simulink model "Sim_Multi"  (R2023a)
settings: Solver=FixedStepAuto  StartTime=0.0  StopTime=20  FixedStep=t_sim  MaxStep=t_control  RelTol=1e-5  EnableMultiTasking=on
InitFcn:
  | %--------------------------------------------------------------------------
  | %% Multirotor Dynamic Simulation Environment for the Testing of GNC Algorithms
  | % This simulation is part of the Master's thesis titled
  | % "A Modular Simulation Environment for the Improved Dynamic Simulation of
  | % Multirotor Unmanned Aerial Vehicles",
  | % submitted to the University of Illinois at Urbana-Champaign in May 2016.
  | % The thesis itself can be found here: http://hdl.handle.net/2142/90660
  | % Jan Vervoorst, vervoors@illinois.edu
  | % University of Illinois 2015/16
  | %--------------------------------------------------------------------------
  | %% Initialization routine for the Simulink simulation file Sim_Multi.slx
  | %--------------------------------------------------------------------------
  | clear all;close all;clc
  | %--------------------------------------------------------------------------
  | t_control = 1/500;          % Controller/state estimation frequency 500Hz [s]
  | t_sim = t_control/2;        % Simulation frequency 1000Hz [s]
  | sim_time = 10.0;            % Duration of simulation [sec]
  | r2d = 180/pi;               % Conversion factor radians to degrees [deg/rad]
  | d2r = pi/180;               % Conversion factor degrees to radians [rad/deg]
  | g = 9.80665;                % Acceleration of gravity [m/s^2]
  | rpm2radpersec = 2*pi/60;    % Conversion factor RPM to rad/sec [rad/(s*rpm)]
  | rho = 1.225;                % Density of air [kg/m^3]
  | %--------------------------------------------------------------------------
  | %%%%%%%%%%%%%%%%%%%%%%%%%%%%%%%%%%%%%%%%%%%%%%%%%%%%%%%%%%%%%%%%%%%%%%%%%%%
  | %               Quad specific configuration parameters                    %
  | %%%%%%%%%%%%%%%%%%%%%%%%%%%%%%%%%%%%%%%%%%%%%%%%%%%%%%%%%%%%%%%%%%%%%%%%%%%
  | % The coordinate system used in this model is defined as follows:
  | % X: pointing forward, Roll axis
  | % Y: pointing to the right, Pitch axis
  | % Z: pointing down, Yaw axis
  | % To define the geometry of the airframe, the following convention is used:
  | % - the base airframe is assumed to be somewhat symmetric
  | % - the CoG for the base airframe coincides with the geometric center in X/Y plane (but is shifted along Z axis)
  | % - the motor arm length in X/Y plane is defined as the distance to the geometric center of the base airframe
  | % - motor thrust is generated at the prop, which is offset a distance (along Z) from the geometric center
  | % - motor thrust vector may be misaligned from purely Z direction, so a set of rotation angles is given for each motor
  | % - real position of CoG is given as a position vector from geometric center
  | % - everything is expressed in body coordinate system described above
  | %%%%%%%%%%%%%%%%%%%%%%%%%%%%%%%%%%%%%%%%%%%%%%%%%%%%%%%%%%%%%%%%%%%%%%%%%%%
  | Noise_flag = 0;                 % Set to 1 for sensor/estimation noise, to 0 for no noise
  | Coriolis_correction = 1;        % Set to 1 to cancel omega x (J*omega) term in control law, 0 if not
  | Dyn_thrust = 1;                 % Set to 1 to engage dynamic thrust effects, to 0 to disengage
  | Blade_flapping = 1;             % Set to 1 to engage blade flapping effects, to 0 to disengage
  | %%%%%%%%%%%%%%%%%%%%%%%%%%%%%%%%
  | % Initial conditions
  | Att_init = [0;0;0] * d2r;       % Initial airframe attitude in Euler angles Roll/Pitch/Yaw for 6DOF block [deg]
  | omega_init = [0;0;0];           % Initial angular rates in Body frame for 6DOF block [rad/s]
  | Vb_init = [0;0;0];              % Initial velocity in Body frame for 6DOF block [m/s]
  | Xi_init = [0;0;0];              % Initial position in Inertial frame for 6DOF block [m]
  | rpm_init = 3104.5025852;        % Initial motor speed [rpm]
  | q_init = rpy2quat(Att_init);    % Compute the initial attitude quaternion
  | R_IB_init = rpy2rot(Att_init);  % Compute the initial rotation matrix R_IB
  | Vi_init = R_IB_init' * Vb_init; % Compute the initial velocity in Inertial axes
  | %%%%%%%%%%%%%%%%%%%%%%%%%%%%%%%%
  | % Parameters for aerodynamic drag computation
  | a = 0.060;                      % Surface area of airframe visible along the Body x axis [m^2]
  | b = 0.060;                      % Surface area of airframe visible along the Body y axis [m^2]
  | c = 0.060;                      % Surface area of airframe visible along the Body z axis [m^2]
  | C_D = 0.40;                     % Drag coefficient [dimensionless]
  | Surface_params = [a;b;c];       % Combine the surface area parameters
  | ... (+145 lines)
undefined symbols (not defined in the file or in its folder): DiscIntNeverNeededParam, rpy2quat, thrust2rpm
libraries: simulink x20
(part 3 of 4)

== system Sim_Multi/multirotor/Force//Moment computation/Forces and moments generated by spinning propellers/For Each Subsystem/Leverarm vector from real CoG to each propeller (Body axes) ==
  note: This subsystem computes the leverarm vector from the real center of gravity
      | of the airframe to each propeller.
      | This vector is necessary to compute the moment contributions of each propeller.
  MotorMatrix_real : Inport
  CoG_real : Inport  Port=2
  Abs : Abs  SaturateOnIntegerOverflow=off
  Conversion deg to rad : Gain  Gain=d2r
  Mux : Mux  Inputs=2
  Mux2 : Mux  Inputs=2
  Product4 : Product
  Reshape : Reshape  OutputDimensionality=Column vector (2-D)
  Reshape1 : Reshape  OutputDimensionality=Column vector (2-D)
  Selector3 : Selector  InputPortWidth=17  IndexOptions=Index vector (dialog)  Indices=[1]  OutputSizes=1
  Selector4 : Selector  InputPortWidth=17  IndexOptions=Index vector (dialog)  Indices=[2]  OutputSizes=1
  Selector5 : Selector  InputPortWidth=17  IndexOptions=Index vector (dialog)  Indices=[3]  OutputSizes=1
  Subtract : Sum  Inputs=+-
  Trigonometric Function : Trigonometry
  Trigonometric Function1 : Trigonometry  Operator=cos
  Prop_vector : Outport
  wires:
  Selector3/1 -> Conversion deg to rad/1  "Motor arm angle"
  Selector4/1 -> Abs/1  "Motor arm length"
  Selector5/1 -> Mux2/2  "Propeller Z offset"
  Conversion deg to rad/1 -> Trigonometric Function/1, Trigonometric Function1/1
  Trigonometric Function1/1 -> Mux/1  "Motor arm x component"
  Trigonometric Function/1 -> Mux/2  "Motor arm y component"
  Mux/1 -> Product4/1
  Abs/1 -> Product4/2
  Product4/1 -> Mux2/1  "Motor location x/y vector"
  Mux2/1 -> Reshape/1
  CoG_real/1 -> Reshape1/1  "Location of real CoG w.r.t. geometric center (Body axes)"
  Reshape/1 -> Subtract/1  "Vector from geometric center to propeller (Body axes)"
  Reshape1/1 -> Subtract/2
  Subtract/1 -> Prop_vector/1  "Vector from real CoG to propeller (Body axes)"
  MotorMatrix_real/1 -> Selector5/1, Selector4/1, Selector3/1

== system Sim_Multi/multirotor/Force//Moment computation/Forces and moments generated by spinning propellers/For Each Subsystem/Thrust//moment vector for each propeller (Body axes) ==
  Prop_vector : Inport
  True airspeed : Inport  Port=2
  Body_rates : Inport  Port=3
  MotorMatrix_real : Inport  Port=4
  RPM_motor : Inport  Port=5
  Add : Sum  Inputs=++++
  Compute dynamic motor thrust and moments : Subsystem
  Coordinate transformation Body to Motor axes : Subsystem
  Cross Product : Subsystem
  Reshape : Reshape  OutputDimensionality=Column vector (2-D)
  Thrust_vector (Body axes) : Outport
  Motor_moments (Body axes) : Outport  Port=2
  wires:
  MotorMatrix_real/1 -> Coordinate transformation Body to Motor axes/1(MotorMatrix_real), Compute dynamic motor thrust and moments/2(MotorMatrix_real)
  True airspeed/1 -> Coordinate transformation Body to Motor axes/2(Airspeed (Body axes))
  Coordinate transformation Body to Motor axes/2(Airspeed (Motor axes)) -> Compute dynamic motor thrust and moments/4(Airspeed (Motor axes))
  RPM_motor/1 -> Compute dynamic motor thrust and moments/1(RPM_motor)
  Body_rates/1 -> Compute dynamic motor thrust and moments/5(Body_rates)
  Compute dynamic motor thrust and moments/3(Gyro moment (Body axes)) -> Add/3  "Gyroscopic moments per motor (Body axes)"
  Compute dynamic motor thrust and moments/1(Induced motor moment (Body axes)) -> Add/1  "Induced motor moment at dynamic conditions (Body axes)"
  Add/1 -> Motor_moments (Body axes)/1
  Coordinate transformation Body to Motor axes/1(R_mb) -> Compute dynamic motor thrust and moments/3(R_mb)
  Compute dynamic motor thrust and moments/4(Thrust_vector (Body axes)) -> Thrust_vector (Body axes)/1, Cross Product/2(v)
  Compute dynamic motor thrust and moments/2(Motor hub moment (Body axes)) -> Add/2  "Moment induced in motor hub due to blade flapping (Body axes)"
  Cross Product/1(u x v) -> Reshape/1
  Prop_vector/1 -> Cross Product/1(u)
  Reshape/1 -> Add/4

== system Sim_Multi/multirotor/Force//Moment computation/Forces and moments generated by spinning propellers/Total airspeed (Body axes)/Inertial to Body ==
  DCM_ib : Inport
  Wind_i : Inport  Port=2
  Product : Product  Multiplication=Matrix(*)
  Reshape : Reshape  OutputDimensionality=Column vector (2-D)
  Reshape1 : Reshape  OutputDimensionality=Column vector (2-D)
  Wind_b : Outport
  wires:
  Reshape/1 -> Product/2
  Product/1 -> Reshape1/1
  Reshape1/1 -> Wind_b/1
  Wind_i/1 -> Reshape/1
  DCM_ib/1 -> Product/1  "DCM_ib"

== system Sim_Multi/Controller/Controller Structure/Inner-loop control only/PI Rate controller/Cross Product/Subsystem ==
  u : Inport
  v : Inport  Port=2
  Demux : Demux  Outputs=3
  Demux1 : Demux  Outputs=3
  Mux : Mux  Inputs=3
  Product : Product
  Product1 : Product
  Product2 : Product
  Positive elements : Outport
  wires:
  Mux/1 -> Positive elements/1
  v/1 -> Demux1/1
  u/1 -> Demux/1
  Demux/2 -> Product/1
  Demux1/3 -> Product/2
  Demux/3 -> Product1/1
  Demux1/1 -> Product1/2
  Demux/1 -> Product2/1
  Demux1/2 -> Product2/2
  Product/1 -> Mux/1
  Product1/1 -> Mux/2
  Product2/1 -> Mux/3

== system Sim_Multi/Controller/Controller Structure/Inner-loop control only/PI Rate controller/Cross Product/Subsystem1 ==
  u : Inport
  v : Inport  Port=2
  Demux : Demux  Outputs=3
  Demux1 : Demux  Outputs=3
  Mux : Mux  Inputs=3
  Product : Product
  Product1 : Product
  Product2 : Product
  Negative elements : Outport
  wires:
  Mux/1 -> Negative elements/1
  v/1 -> Demux1/1
  u/1 -> Demux/1
  Product/1 -> Mux/1
  Product1/1 -> Mux/2
  Product2/1 -> Mux/3
  Demux/3 -> Product/1
  Demux1/2 -> Product/2
  Demux/1 -> Product1/1
  Demux1/3 -> Product1/2
  Demux/2 -> Product2/1
  Demux1/1 -> Product2/2

== system Sim_Multi/Controller/Controller Structure/Inner-loop control only/PI Rate controller/Gain Kff/Create diagonal 3x3 matrix ==
  Vector : Inport
  Constant2 : Constant  Value=0
  Demux : Demux  Outputs=3
  Subsystem9 : Subsystem
  Matrix : Outport
  wires:
  Demux/1 -> Subsystem9/1(C_11)
  Demux/2 -> Subsystem9/5(C_22)
  Vector/1 -> Demux/1
  Constant2/1 -> Subsystem9/8(C_32), Subsystem9/7(C_31), Subsystem9/6(C_23), Subsystem9/4(C_21), Subsystem9/3(C_13), Subsystem9/2(C_12)
  Subsystem9/1(Diag) -> Matrix/1
  Demux/3 -> Subsystem9/9(C_33)

== system Sim_Multi/Controller/Controller Structure/Inner-loop control only/PI Rate controller/Gain Ki/Create diagonal 3x3 matrix ==
  Vector : Inport
  Constant2 : Constant  Value=0
  Demux : Demux  Outputs=3
  Subsystem9 : Subsystem
  Matrix : Outport
  wires:
  Demux/1 -> Subsystem9/1(C_11)
  Demux/2 -> Subsystem9/5(C_22)
  Vector/1 -> Demux/1
  Constant2/1 -> Subsystem9/8(C_32), Subsystem9/7(C_31), Subsystem9/6(C_23), Subsystem9/4(C_21), Subsystem9/3(C_13), Subsystem9/2(C_12)
  Subsystem9/1(Diag) -> Matrix/1
  Demux/3 -> Subsystem9/9(C_33)

== system Sim_Multi/Controller/Controller Structure/Inner-loop control only/PI Rate controller/Gain Kp/Create diagonal 3x3 matrix ==
  Vector : Inport
  Constant2 : Constant  Value=0
  Demux : Demux  Outputs=3
  Subsystem9 : Subsystem
  Matrix : Outport
  wires:
  Demux/1 -> Subsystem9/1(C_11)
  Demux/2 -> Subsystem9/5(C_22)
  Vector/1 -> Demux/1
  Constant2/1 -> Subsystem9/8(C_32), Subsystem9/7(C_31), Subsystem9/6(C_23), Subsystem9/4(C_21), Subsystem9/3(C_13), Subsystem9/2(C_12)
  Subsystem9/1(Diag) -> Matrix/1
  Demux/3 -> Subsystem9/9(C_33)

== system Sim_Multi/multirotor/6DOF model/Quat Strapdown Eq./Normalize/norm/dot_product ==
  u : Inport
  v : Inport  Port=2
  Product : Product  Multiplication=Matrix(*)  RndMeth=Zero
  Reshape : Reshape  OutputDimensionality=Column vector (2-D)
  Reshape1 : Reshape  OutputDimensionality=Column vector (2-D)
  transpose : Math  Operator=transpose  SignedPower=on
  u.v : Outport
  wires:
  v/1 -> Reshape1/1
  u/1 -> Reshape/1
  Reshape/1 -> transpose/1
  transpose/1 -> Product/1
  Reshape1/1 -> Product/2
  Product/1 -> u.v/1

== system Sim_Multi/multirotor/Force//Moment computation/Compute aerodynamic drag of the airframe in Body axes/Aerodynamic drag force/Nonzero airspeed/Normalize ==
  Input : Inport
  Divide : Product  Inputs=*/
  norm : Subsystem
  Output : Outport
  wires:
  Input/1 -> Divide/1, norm/1(u)
  norm/1(||u||) -> Divide/2
  Divide/1 -> Output/1

== system Sim_Multi/multirotor/Force//Moment computation/Compute aerodynamic drag of the airframe in Body axes/Aerodynamic drag force/Nonzero airspeed/Surface area computation ==
  Airspeed (Body) : Inport
  Surface_params : Inport  Port=2
  Scaling factor computation : Subsystem
  Surface area computation : Subsystem
  Area : Outport
  wires:
  Surface_params/1 -> Scaling factor computation/2(Surface_params)
  Airspeed (Body)/1 -> Surface area computation/1(Airspeed (Body)), Scaling factor computation/1(Airspeed (Body))
  Scaling factor computation/1(Scaling factor) -> Surface area computation/2(Scaling factor)
  Surface area computation/1(Surface area) -> Area/1

== system Sim_Multi/multirotor/Force//Moment computation/Compute aerodynamic drag of the airframe in Body axes/Aerodynamic drag force/Nonzero airspeed/u^2 ==
  u : Inport
  dot_product : Subsystem
  u^2 : Outport
  wires:
  u/1 -> dot_product/1(u), dot_product/2(v)
  dot_product/1(u.v) -> u^2/1

== system Sim_Multi/multirotor/Force//Moment computation/Compute aerodynamic drag of the airframe in Body axes/Aerodynamic drag force/norm/dot_product ==
  u : Inport
  v : Inport  Port=2
  Product : Product  Multiplication=Matrix(*)  RndMeth=Zero
  Reshape : Reshape  OutputDimensionality=Column vector (2-D)
  Reshape1 : Reshape  OutputDimensionality=Column vector (2-D)
  transpose : Math  Operator=transpose  SignedPower=on
  u.v : Outport
  wires:
  v/1 -> Reshape1/1
  u/1 -> Reshape/1
  Reshape/1 -> transpose/1
  transpose/1 -> Product/1
  Reshape1/1 -> Product/2
  Product/1 -> u.v/1

== system Sim_Multi/multirotor/Force//Moment computation/Forces and moments generated by spinning propellers/For Each Subsystem/Actuator dynamics/Continuous Integrator with dynamic upper//lower limits ==
  Integrator input : Inport
  Lower limit : Inport  Port=2
  Upper limit : Inport  Port=3
  Compare To Zero : simulink/Logic and Bit Operations/Compare To Zero  relop=<  OutDataTypeStr=uint8  ZeroCross=off
  Compare To Zero1 : simulink/Logic and Bit Operations/Compare To Zero  relop=>  OutDataTypeStr=uint8  ZeroCross=off
  Constant : Constant  Value=0
  Integrator : Integrator  InitialCondition=rpm_init
  Logical Operator : Logic  Operator=OR  AllPortsSameDT=off  OutDataTypeStr=boolean
  Logical Operator1 : Logic  Operator=OR  AllPortsSameDT=off  OutDataTypeStr=boolean
  Logical Operator2 : Logic  AllPortsSameDT=off  OutDataTypeStr=boolean
  Relational Operator : RelationalOperator  Operator=<=  OutDataTypeStr=boolean  InputSameDT=off
  Relational Operator1 : RelationalOperator  OutDataTypeStr=boolean  InputSameDT=off
  Saturation Dynamic : simulink/Discontinuities/Saturation Dynamic  OutMin=[]  OutMax=[]  OutDataTypeStr=Inherit: Same as second input  OutDataType=fixdt(1, 16)  OutScaling=2^-10  DoSatur=off
  Switch : Switch  Criteria=u2 > Threshold  SaturateOnIntegerOverflow=off  InputSameDT=off
  Output : Outport
  wires:
  Integrator input/1 -> Switch/1, Compare To Zero1/1, Compare To Zero/1
  Constant/1 -> Switch/3
  Switch/1 -> Integrator/1
  Relational Operator/1 -> Logical Operator/1
  Compare To Zero/1 -> Logical Operator/2
  Upper limit/1 -> Relational Operator/2, Saturation Dynamic/1
  Lower limit/1 -> Saturation Dynamic/3, Relational Operator1/2
  Compare To Zero1/1 -> Logical Operator1/1
  Relational Operator1/1 -> Logical Operator1/2
  Logical Operator1/1 -> Logical Operator2/2
  Logical Operator/1 -> Logical Operator2/1
  Logical Operator2/1 -> Switch/2
  Saturation Dynamic/1 -> Output/1
  Integrator/1 -> Relational Operator/1, Saturation Dynamic/2, Relational Operator1/1

== system Sim_Multi/multirotor/Force//Moment computation/Forces and moments generated by spinning propellers/For Each Subsystem/Actuator dynamics/Continuous Integrator with dynamic upper//lower limits1 ==
  Integrator input : Inport
  Lower limit : Inport  Port=2
  Upper limit : Inport  Port=3
  Compare To Zero : simulink/Logic and Bit Operations/Compare To Zero  relop=<  OutDataTypeStr=uint8  ZeroCross=off
  Compare To Zero1 : simulink/Logic and Bit Operations/Compare To Zero  relop=>  OutDataTypeStr=uint8  ZeroCross=off
  Constant : Constant  Value=0
  Integrator : Integrator  InitialCondition=rpm_init
  Logical Operator : Logic  Operator=OR  AllPortsSameDT=off  OutDataTypeStr=boolean
  Logical Operator1 : Logic  Operator=OR  AllPortsSameDT=off  OutDataTypeStr=boolean
  Logical Operator2 : Logic  AllPortsSameDT=off  OutDataTypeStr=boolean
  Relational Operator : RelationalOperator  Operator=<=  OutDataTypeStr=boolean  InputSameDT=off
  Relational Operator1 : RelationalOperator  OutDataTypeStr=boolean  InputSameDT=off
  Saturation Dynamic : simulink/Discontinuities/Saturation Dynamic  OutMin=[]  OutMax=[]  OutDataTypeStr=Inherit: Same as second input  OutDataType=fixdt(1, 16)  OutScaling=2^-10  DoSatur=off
  Switch : Switch  Criteria=u2 > Threshold  SaturateOnIntegerOverflow=off  InputSameDT=off
  Output : Outport
  wires:
  Integrator/1 -> Relational Operator1/1, Saturation Dynamic/2, Relational Operator/1
  Saturation Dynamic/1 -> Output/1
  Logical Operator2/1 -> Switch/2
  Logical Operator/1 -> Logical Operator2/1
  Logical Operator1/1 -> Logical Operator2/2
  Relational Operator1/1 -> Logical Operator1/2
  Compare To Zero1/1 -> Logical Operator1/1
  Lower limit/1 -> Relational Operator1/2, Saturation Dynamic/3
  Upper limit/1 -> Saturation Dynamic/1, Relational Operator/2
  Compare To Zero/1 -> Logical Operator/2
  Relational Operator/1 -> Logical Operator/1
  Switch/1 -> Integrator/1
  Constant/1 -> Switch/3
  Integrator input/1 -> Compare To Zero/1, Compare To Zero1/1, Switch/1

== system Sim_Multi/multirotor/Force//Moment computation/Forces and moments generated by spinning propellers/For Each Subsystem/Cross Product/Subsystem ==
  omega : Inport
  r : Inport  Port=2
  Demux : Demux  Outputs=3
  Demux1 : Demux  Outputs=3
  Mux : Mux  Inputs=3
  Product : Product
  Product1 : Product
  Product2 : Product
  Positive elements : Outport
  wires:
  Mux/1 -> Positive elements/1
  r/1 -> Demux1/1
  omega/1 -> Demux/1
  Demux/2 -> Product/1
  Demux1/3 -> Product/2
  Demux/3 -> Product1/1
  Demux1/1 -> Product1/2
  Demux/1 -> Product2/1
  Demux1/2 -> Product2/2
  Product/1 -> Mux/1  "u2*v3"
  Product1/1 -> Mux/2  "u3*v1"
  Product2/1 -> Mux/3  "u1*v2"

== system Sim_Multi/multirotor/Force//Moment computation/Forces and moments generated by spinning propellers/For Each Subsystem/Cross Product/Subsystem1 ==
  omega : Inport
  r : Inport  Port=2
  Demux : Demux  Outputs=3
  Demux1 : Demux  Outputs=3
  Mux : Mux  Inputs=3
  Product : Product
  Product1 : Product
  Product2 : Product
  Negative elements : Outport
  wires:
  Mux/1 -> Negative elements/1
  r/1 -> Demux1/1
  omega/1 -> Demux/1
  Product/1 -> Mux/1  "u3*v2"
  Product1/1 -> Mux/2  "u1*v3"
  Product2/1 -> Mux/3  "u2*v1"
  Demux/3 -> Product/1
  Demux1/2 -> Product/2
  Demux/1 -> Product1/1
  Demux1/3 -> Product1/2
  Demux/2 -> Product2/1
  Demux1/1 -> Product2/2

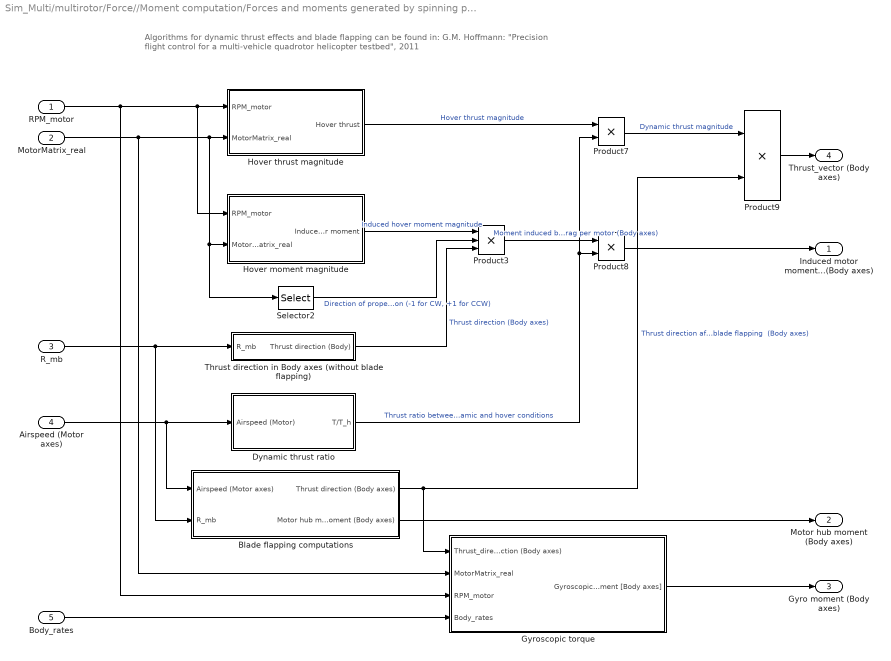
== system Sim_Multi/multirotor/Force//Moment computation/Forces and moments generated by spinning propellers/For Each Subsystem/Thrust//moment vector for each propeller (Body axes)/Compute dynamic motor thrust and moments ==
  note: Algorithms for dynamic thrust effects and blade flapping can be found in:
      | G.M. Hoffmann: "Precision flight control for a multi-vehicle quadrotor helicopter testbed", 2011
  RPM_motor : Inport
  MotorMatrix_real : Inport  Port=2
  R_mb : Inport  Port=3
  Airspeed (Motor axes) : Inport  Port=4
  Body_rates : Inport  Port=5
  Blade flapping computations : Subsystem
  Dynamic thrust ratio : Subsystem
  Gyroscopic torque : Subsystem
  Hover moment magnitude : Subsystem
  Hover thrust magnitude : Subsystem
  Product3 : Product  Inputs=3
  Product7 : Product
  Product8 : Product
  Product9 : Product
  Selector2 : Selector  InputPortWidth=17  IndexOptions=Index vector (dialog)  Indices=[4]  OutputSizes=1
  Thrust direction in Body axes (without blade flapping) : Subsystem
  Induced motor moment (Body axes) : Outport
  Motor hub moment (Body axes) : Outport  Port=2
  Gyro moment (Body axes) : Outport  Port=3
  Thrust_vector (Body axes) : Outport  Port=4
  wires:
  RPM_motor/1 -> Gyroscopic torque/3(RPM_motor), Hover moment magnitude/1(RPM_motor), Hover thrust magnitude/1(RPM_motor)
  MotorMatrix_real/1 -> Gyroscopic torque/2(MotorMatrix_real), Selector2/1, Hover moment magnitude/2(MotorMatrix_real), Hover thrust magnitude/2(MotorMatrix_real)
  Selector2/1 -> Product3/2  "Direction of propeller rotation (-1 for CW, +1 for CCW)"
  Thrust direction in Body axes (without blade flapping)/1(Thrust direction (Body)) -> Product3/3  "Thrust direction (Body axes)"
  R_mb/1 -> Blade flapping computations/2(R_mb), Thrust direction in Body axes (without blade flapping)/1(R_mb)
  Airspeed (Motor axes)/1 -> Blade flapping computations/1(Airspeed (Motor axes)), Dynamic thrust ratio/1(Airspeed (Motor))
  Product3/1 -> Product8/1  "Moment induced by aerodynamic drag per motor (Body axes)"
  Product8/1 -> Induced motor moment (Body axes)/1
  Product7/1 -> Product9/1  "Dynamic thrust magnitude"
  Product9/1 -> Thrust_vector (Body axes)/1
  Blade flapping computations/1(Thrust direction (Body axes)) -> Gyroscopic torque/1(Thrust_direction (Body axes)), Product9/2  "Thrust direction after blade flapping  (Body axes)"
  Blade flapping computations/2(Motor hub moment (Body axes)) -> Motor hub moment (Body axes)/1
  Body_rates/1 -> Gyroscopic torque/4(Body_rates)
  Gyroscopic torque/1(Gyroscopic moment [Body axes]) -> Gyro moment (Body axes)/1
  Hover thrust magnitude/1(Hover thrust) -> Product7/1  "Hover thrust magnitude"
  Hover moment magnitude/1(Induced hover moment) -> Product3/1  "Induced hover moment magnitude"
  Dynamic thrust ratio/1(T/T_h) -> Product7/2, Product8/2  "Thrust ratio between dynamic and hover conditions"

== system Sim_Multi/multirotor/Force//Moment computation/Forces and moments generated by spinning propellers/For Each Subsystem/Thrust//moment vector for each propeller (Body axes)/Coordinate transformation Body to Motor axes ==
  note: The true airspeed at prop computed here is the linear velocity (now in Motor axes)
      | with which this particular motor moves through the air.
      | So the point of view is: the surrounding air standing still and the airframe moving through it.
  MotorMatrix_real : Inport
  Airspeed (Body axes) : Inport  Port=2
  Conversion deg to rad : Gain  Gain=d2r
  Product : Product  Multiplication=Matrix(*)
  Rotation Matrix Body to Motor : Subsystem
  Selector : Selector  InputPortWidth=17  IndexOptions=Index vector (dialog)  Indices=[13 14 15]  OutputSizes=1
  R_mb : Outport
  Airspeed (Motor axes) : Outport  Port=2
  wires:
  Product/1 -> Airspeed (Motor axes)/1  "True airspeed at prop (Motor axes)"
  Rotation Matrix Body to Motor/1(R_mb) -> R_mb/1, Product/1  "Rotation matrix Body to Motor axes"
  MotorMatrix_real/1 -> Selector/1
  Selector/1 -> Conversion deg to rad/1
  Airspeed (Body axes)/1 -> Product/2  "True airspeed at prop (Body axes)"
  Conversion deg to rad/1 -> Rotation Matrix Body to Motor/1(Motor angles)

== system Sim_Multi/multirotor/Force//Moment computation/Forces and moments generated by spinning propellers/For Each Subsystem/Thrust//moment vector for each propeller (Body axes)/Cross Product ==
  u : Inport
  v : Inport  Port=2
  Subsystem : Subsystem
  Subsystem1 : Subsystem
  Sum : Sum  Inputs=+|-
  u x v : Outport
  wires:
  Sum/1 -> u x v/1
  u/1 -> Subsystem1/1(u), Subsystem/1(u)
  v/1 -> Subsystem1/2(v), Subsystem/2(v)
  Subsystem/1(Positive elements) -> Sum/1
  Subsystem1/1(Negative elements) -> Sum/2

== system Sim_Multi/Controller/Controller Structure/Inner-loop control only/PI Rate controller/Gain Kff/Create diagonal 3x3 matrix/Subsystem9 ==
  C_11 : Inport  PortDimensions=1
  C_12 : Inport  Port=2  PortDimensions=1
  C_13 : Inport  Port=3  PortDimensions=1
  C_21 : Inport  Port=4  PortDimensions=1
  C_22 : Inport  Port=5  PortDimensions=1
  C_23 : Inport  Port=6  PortDimensions=1
  C_31 : Inport  Port=7  PortDimensions=1
  C_32 : Inport  Port=8  PortDimensions=1
  C_33 : Inport  Port=9  PortDimensions=1
  Reshape (9) to [3x3] column-major : Reshape  OutputDimensionality=Customize  OutputDimensions=[3,3]
  Vector Concatenate : Concatenate  NumInputs=9
  Diag : Outport
  wires:
  C_33/1 -> Vector Concatenate/9
  C_22/1 -> Vector Concatenate/5
  Reshape (9) to [3x3] column-major/1 -> Diag/1
  C_11/1 -> Vector Concatenate/1
  Vector Concatenate/1 -> Reshape (9) to [3x3] column-major/1
  C_32/1 -> Vector Concatenate/6
  C_31/1 -> Vector Concatenate/3
  C_21/1 -> Vector Concatenate/2
  C_13/1 -> Vector Concatenate/7
  C_12/1 -> Vector Concatenate/4
  C_23/1 -> Vector Concatenate/8

== system Sim_Multi/Controller/Controller Structure/Inner-loop control only/PI Rate controller/Gain Ki/Create diagonal 3x3 matrix/Subsystem9 ==
  C_11 : Inport  PortDimensions=1
  C_12 : Inport  Port=2  PortDimensions=1
  C_13 : Inport  Port=3  PortDimensions=1
  C_21 : Inport  Port=4  PortDimensions=1
  C_22 : Inport  Port=5  PortDimensions=1
  C_23 : Inport  Port=6  PortDimensions=1
  C_31 : Inport  Port=7  PortDimensions=1
  C_32 : Inport  Port=8  PortDimensions=1
  C_33 : Inport  Port=9  PortDimensions=1
  Reshape (9) to [3x3] column-major : Reshape  OutputDimensionality=Customize  OutputDimensions=[3,3]
  Vector Concatenate : Concatenate  NumInputs=9
  Diag : Outport
  wires:
  C_33/1 -> Vector Concatenate/9
  C_22/1 -> Vector Concatenate/5
  Reshape (9) to [3x3] column-major/1 -> Diag/1
  C_11/1 -> Vector Concatenate/1
  Vector Concatenate/1 -> Reshape (9) to [3x3] column-major/1
  C_32/1 -> Vector Concatenate/6
  C_31/1 -> Vector Concatenate/3
  C_21/1 -> Vector Concatenate/2
  C_13/1 -> Vector Concatenate/7
  C_12/1 -> Vector Concatenate/4
  C_23/1 -> Vector Concatenate/8

== system Sim_Multi/Controller/Controller Structure/Inner-loop control only/PI Rate controller/Gain Kp/Create diagonal 3x3 matrix/Subsystem9 ==
  C_11 : Inport  PortDimensions=1
  C_12 : Inport  Port=2  PortDimensions=1
  C_13 : Inport  Port=3  PortDimensions=1
  C_21 : Inport  Port=4  PortDimensions=1
  C_22 : Inport  Port=5  PortDimensions=1
  C_23 : Inport  Port=6  PortDimensions=1
  C_31 : Inport  Port=7  PortDimensions=1
  C_32 : Inport  Port=8  PortDimensions=1
  C_33 : Inport  Port=9  PortDimensions=1
  Reshape (9) to [3x3] column-major : Reshape  OutputDimensionality=Customize  OutputDimensions=[3,3]
  Vector Concatenate : Concatenate  NumInputs=9
  Diag : Outport
  wires:
  C_33/1 -> Vector Concatenate/9
  C_22/1 -> Vector Concatenate/5
  Reshape (9) to [3x3] column-major/1 -> Diag/1
  C_11/1 -> Vector Concatenate/1
  Vector Concatenate/1 -> Reshape (9) to [3x3] column-major/1
  C_32/1 -> Vector Concatenate/6
  C_31/1 -> Vector Concatenate/3
  C_21/1 -> Vector Concatenate/2
  C_13/1 -> Vector Concatenate/7
  C_12/1 -> Vector Concatenate/4
  C_23/1 -> Vector Concatenate/8

== system Sim_Multi/multirotor/Force//Moment computation/Compute aerodynamic drag of the airframe in Body axes/Aerodynamic drag force/Nonzero airspeed/Normalize/norm ==
  u : Inport
  Complex to Real-Imag : ComplexToRealImag  Output=Real
  Sqrt : Sqrt
  dot_product : Subsystem
  ||u|| : Outport
  wires:
  u/1 -> dot_product/1(u), dot_product/2(v)
  dot_product/1(u.v) -> Sqrt/1
  Sqrt/1 -> Complex to Real-Imag/1
  Complex to Real-Imag/1 -> ||u||/1

== system Sim_Multi/multirotor/Force//Moment computation/Compute aerodynamic drag of the airframe in Body axes/Aerodynamic drag force/Nonzero airspeed/Surface area computation/Scaling factor computation ==
  Airspeed (Body) : Inport
  Surface_params : Inport  Port=2
  Add : Sum  Inputs=+++
  Demux : Demux  Outputs=3
  Demux1 : Demux  Outputs=3
  Divide : Product  Inputs=*/
  Divide1 : Product  Inputs=*/
  Divide2 : Product  Inputs=*/
  Product : Product
  Product1 : Product
  Product2 : Product
  Reciprocal Sqrt : Sqrt  Operator=rSqrt
  Scaling factor : Outport
  wires:
  Divide2/1 -> Product2/2, Product2/1
  Reciprocal Sqrt/1 -> Scaling factor/1
  Demux1/3 -> Divide2/2  "c"
  Demux/3 -> Divide2/1  "z"
  Divide/1 -> Product/2, Product/1
  Airspeed (Body)/1 -> Demux/1
  Surface_params/1 -> Demux1/1
  Demux1/1 -> Divide/2  "a"
  Demux/1 -> Divide/1  "x"
  Product/1 -> Add/1
  Product2/1 -> Add/3
  Add/1 -> Reciprocal Sqrt/1
  Demux/2 -> Divide1/1  "y"
  Divide1/1 -> Product1/2, Product1/1
  Demux1/2 -> Divide1/2  "b"
  Product1/1 -> Add/2

== system Sim_Multi/multirotor/Force//Moment computation/Compute aerodynamic drag of the airframe in Body axes/Aerodynamic drag force/Nonzero airspeed/Surface area computation/Surface area computation ==
  Airspeed (Body) : Inport
  Scaling factor : Inport  Port=2
  Product : Product
  norm : Subsystem
  Surface area : Outport
  wires:
  Scaling factor/1 -> Product/2
  Airspeed (Body)/1 -> Product/1
  Product/1 -> norm/1(u)
  norm/1(||u||) -> Surface area/1

== system Sim_Multi/multirotor/Force//Moment computation/Compute aerodynamic drag of the airframe in Body axes/Aerodynamic drag force/Nonzero airspeed/u^2/dot_product ==
  u : Inport
  v : Inport  Port=2
  Product : Product  Multiplication=Matrix(*)  RndMeth=Zero
  Reshape : Reshape  OutputDimensionality=Column vector (2-D)
  Reshape1 : Reshape  OutputDimensionality=Column vector (2-D)
  transpose : Math  Operator=transpose  SignedPower=on
  u.v : Outport
  wires:
  v/1 -> Reshape1/1
  u/1 -> Reshape/1
  Reshape/1 -> transpose/1
  transpose/1 -> Product/1
  Reshape1/1 -> Product/2
  Product/1 -> u.v/1

== system Sim_Multi/multirotor/Force//Moment computation/Forces and moments generated by spinning propellers/For Each Subsystem/Thrust//moment vector for each propeller (Body axes)/Compute dynamic motor thrust and moments/Blade flapping computations ==
  note: Blade flapping computations are motivated by algorithms found in:
      | G.M. Hoffmann: "Precision flight control for a multi-vehicle quadrotor helicopter testbed", 2011
      | The idea is the following:
      | The thrust vector is tilted backwards from the direction of motion. The amount of tilt depends on the magnitude of the airspeed vector in the (untilted) propeller plane.
      | The tilt direction is in the plane defined by the airspeed xy vector and the (untilted) thrust vector in Motor axes.
      | The normal vector to this plane can be found by computing the cross product of untilted thrust vector and airspeed xy vector.
      | The new (tilted) thrust vector can then be found by applying the Rodrigues rotation formula, see Wikipedia
  Airspeed (Motor axes) : Inport
  R_mb : Inport  Port=2
  Demux4 : Demux  Outputs=[2,1]
  If : If  IfExpression=u1 == 0
  Merge : Merge
  Merge1 : Merge
  Nonzero airspeed in rotor plane : Subsystem  TreatAsAtomicUnit=on
  Terminator : Terminator
  Zero airspeed in rotor plane : Subsystem  TreatAsAtomicUnit=on
  norm : Subsystem
  Thrust direction (Body axes) : Outport
  Motor hub moment (Body axes) : Outport  Port=2
  wires:
  If/1 -> Zero airspeed in rotor plane/Action
  Zero airspeed in rotor plane/1(Thrust direction (Body)) -> Merge/1
  Nonzero airspeed in rotor plane/1(Thrust direction (Body)) -> Merge/2
  If/2 -> Nonzero airspeed in rotor plane/Action
  Airspeed (Motor axes)/1 -> Demux4/1
  Demux4/2 -> Terminator/1  "Airspeed component along motor shaft"
  Demux4/1 -> norm/1(u), Zero airspeed in rotor plane/1(Airspeed xy), Nonzero airspeed in rotor plane/1(Airspeed xy)  "Airspeed components in (unbent) rotor plane"
  norm/1(||u||) -> If/1  "Airspeed xy component  magnitude"
  Merge/1 -> Thrust direction (Body axes)/1  "New tilted thrust direction (Body axes) (This is a unit vector)"
  R_mb/1 -> Nonzero airspeed in rotor plane/2(R_mb), Zero airspeed in rotor plane/2(R_mb)
  Merge1/1 -> Motor hub moment (Body axes)/1  "Moment in the motor hub due to bending of the propeller (Body axes)"
  Zero airspeed in rotor plane/2(Hub moment (Body)) -> Merge1/1
  Nonzero airspeed in rotor plane/2(Hub moment (Body)) -> Merge1/2

== system Sim_Multi/multirotor/Force//Moment computation/Forces and moments generated by spinning propellers/For Each Subsystem/Thrust//moment vector for each propeller (Body axes)/Compute dynamic motor thrust and moments/Dynamic thrust ratio ==
  Airspeed (Motor) : Inport
  Angle of attack and airspeed magnitude : Subsystem
  Compute the climb speed : Subsystem
  Constant : Constant
  Constant1 : Constant  Value=Dyn_thrust
  Divide : Product  Inputs=*/
  Flight modes of the propeller : Subsystem
  Induced velocity at hover : Constant  Value=v_h
  Product2 : Product
  Sum2 : Sum  Inputs=|+-
  Switch : Switch  Criteria=u2 > Threshold  Threshold=0.5  SaturateOnIntegerOverflow=off  InputSameDT=off
  Trigonometric Function : Trigonometry
  T/T_h : Outport
  wires:
  Airspeed (Motor)/1 -> Angle of attack and airspeed magnitude/1(Airspeed (Motor axes)), Compute the climb speed/1(Airspeed (Motor axes))
  Trigonometric Function/1 -> Product2/1
  Sum2/1 -> Divide/2
  Angle of attack and airspeed magnitude/2(Airspeed magnitude) -> Product2/2  "Airspeed magnitude v_inf"
  Angle of attack and airspeed magnitude/1(AoA (rad)) -> Trigonometric Function/1  "Angle of Attack"
  Compute the climb speed/1(v_c) -> Flight modes of the propeller/2(v_c)
  Flight modes of the propeller/1(v_i) -> Sum2/1
  Product2/1 -> Sum2/2
  Induced velocity at hover/1 -> Divide/1, Flight modes of the propeller/1(v_h)
  Switch/1 -> T/T_h/1  "Thrust ratio T/T_h"
  Divide/1 -> Switch/1
  Constant/1 -> Switch/3
  Constant1/1 -> Switch/2

== system Sim_Multi/multirotor/Force//Moment computation/Forces and moments generated by spinning propellers/For Each Subsystem/Thrust//moment vector for each propeller (Body axes)/Compute dynamic motor thrust and moments/Gyroscopic torque ==
  note: The thrust direction chosen here is the one after the effects of blade flapping.
      | The reasoning being that the propeller is bent in that direction and therefore
      | a majority of its moment of inertia effects will act in that direction as well (even
      | though the motor is not affected by blade flapping).
  Thrust_direction (Body axes) : Inport
  MotorMatrix_real : Inport  Port=2
  RPM_motor : Inport  Port=3
  Body_rates : Inport  Port=4
  Conversion rpm to rad/s : Gain  Gain=rpm2radpersec
  Cross Product : Subsystem
  Product5 : Product  Inputs=4
  Propeller moment of inertia : Subsystem
  Reshape1 : Reshape  OutputDimensionality=Column vector (2-D)
  Reshape2 : Reshape  OutputDimensionality=Row vector (2-D)
  Selector6 : Selector  InputPortWidth=17  IndexOptions=Index vector (dialog)  Indices=[4]  OutputSizes=1
  Gyroscopic moment [Body axes] : Outport
  wires:
  Body_rates/1 -> Reshape2/1
  Product5/1 -> Reshape1/1
  Cross Product/1(u x v) -> Product5/3
  Propeller moment of inertia/1(Out1) -> Product5/1  "Moment of inertia for each propeller"
  Selector6/1 -> Product5/2  "Direction of propeller rotation (+1 for CW, -1 for CCW)"
  Conversion rpm to rad/s/1 -> Product5/4
  RPM_motor/1 -> Conversion rpm to rad/s/1
  MotorMatrix_real/1 -> Selector6/1, Propeller moment of inertia/1(In1)
  Thrust_direction (Body axes)/1 -> Cross Product/2(v)  "Thrust direction (Body axes)"
  Reshape2/1 -> Cross Product/1(u)
  Reshape1/1 -> Gyroscopic moment [Body axes]/1

== system Sim_Multi/multirotor/Force//Moment computation/Forces and moments generated by spinning propellers/For Each Subsystem/Thrust//moment vector for each propeller (Body axes)/Compute dynamic motor thrust and moments/Hover moment magnitude ==
  RPM_motor : Inport
  MotorMatrix_real : Inport  Port=2
  Product : Product
  Product1 : Product  Inputs=3
  Selector : Selector  InputPortWidth=17  IndexOptions=Index vector (dialog)  Indices=[9]  OutputSizes=1
  Selector1 : Selector  InputPortWidth=17  IndexOptions=Index vector (dialog)  Indices=[10]  OutputSizes=1
  Sum : Sum  Inputs=|++
  Induced hover moment : Outport
  wires:
  Selector/1 -> Product/2  "Linear torque parameter b1"
  Selector1/1 -> Product1/3  "Quadratic torque parameter b2"
  Product1/1 -> Sum/2
  Product/1 -> Sum/1
  Sum/1 -> Induced hover moment/1  "Motor torque magnitude"
  RPM_motor/1 -> Product/1, Product1/1, Product1/2
  MotorMatrix_real/1 -> Selector1/1, Selector/1

== system Sim_Multi/multirotor/Force//Moment computation/Forces and moments generated by spinning propellers/For Each Subsystem/Thrust//moment vector for each propeller (Body axes)/Compute dynamic motor thrust and moments/Hover thrust magnitude ==
  RPM_motor : Inport
  MotorMatrix_real : Inport  Port=2
  Product4 : Product
  Product5 : Product
  Product6 : Product
  Selector3 : Selector  InputPortWidth=17  IndexOptions=Index vector (dialog)  Indices=[7]  OutputSizes=1
  Selector4 : Selector  InputPortWidth=17  IndexOptions=Index vector (dialog)  Indices=[8]  OutputSizes=1
  Sum1 : Sum  Inputs=|++
  Hover thrust : Outport
  wires:
  Selector4/1 -> Product6/2  "Quadratic thrust parameter a2"
  Selector3/1 -> Product4/2  "Linear thrust parameter a1"
  Product6/1 -> Sum1/2
  Product5/1 -> Product6/1
  Product4/1 -> Sum1/1
  Sum1/1 -> Hover thrust/1  "Hover thrust magnitude"
  MotorMatrix_real/1 -> Selector4/1, Selector3/1
  RPM_motor/1 -> Product4/1, Product5/1, Product5/2

== system Sim_Multi/multirotor/Force//Moment computation/Forces and moments generated by spinning propellers/For Each Subsystem/Thrust//moment vector for each propeller (Body axes)/Compute dynamic motor thrust and moments/Thrust direction in Body axes (without blade flapping) ==
  R_mb : Inport
  Constant : Constant  Value=[0;0;-1]
  Math Function : Math  Operator=transpose  SignedPower=on
  Product9 : Product  Multiplication=Matrix(*)
  Reshape5 : Reshape  OutputDimensionality=Column vector (2-D)
  Thrust direction (Body) : Outport
  wires:
  Reshape5/1 -> Thrust direction (Body)/1
  Product9/1 -> Reshape5/1
  R_mb/1 -> Math Function/1  "Rotation matrix Body to Motor axes"
  Constant/1 -> Product9/2  "Thrust direction vector (Motor axes)"
  Math Function/1 -> Product9/1

== system Sim_Multi/multirotor/Force//Moment computation/Forces and moments generated by spinning propellers/For Each Subsystem/Thrust//moment vector for each propeller (Body axes)/Coordinate transformation Body to Motor axes/Rotation Matrix Body to Motor ==
  note: This is the rotation matrix R_123 as described in:
      | J. Diebel: "Representing Attitude: Euler Angles, Unit Quaternions, and Rotation Vectors", 10/20/2006
  Motor angles : Inport
  Subsystem : Subsystem
  Subsystem1 : Subsystem
  Subsystem2 : Subsystem
  Subsystem3 : Subsystem
  Subsystem4 : Subsystem
  Subsystem5 : Subsystem
  Subsystem6 : Subsystem
  Subsystem7 : Subsystem
  Subsystem8 : Subsystem
  Subsystem9 : Subsystem
  R_mb : Outport
  wires:
  Motor angles/1 -> Subsystem1/1(Euler), Subsystem2/1(Euler), Subsystem3/1(Euler), Subsystem4/1(Euler), Subsystem5/1(Euler), Subsystem6/1(Euler), Subsystem8/1(Euler), Subsystem7/1(Euler), Subsystem/1(Euler)
  Subsystem/1(R_11) -> Subsystem9/1(R_11)
  Subsystem1/1(R_12) -> Subsystem9/2(R_12)
  Subsystem2/1(R_13) -> Subsystem9/3(R_13)
  Subsystem3/1(R_21) -> Subsystem9/4(R_21)
  Subsystem4/1(R_22) -> Subsystem9/5(R_22)
  Subsystem8/1(R_33) -> Subsystem9/9(R_33)
  Subsystem7/1(R_32) -> Subsystem9/8(R_32)
  Subsystem6/1(R_31) -> Subsystem9/7(R_31)
  Subsystem5/1(R_23) -> Subsystem9/6(R_23)
  Subsystem9/1(R_mb) -> R_mb/1

== system Sim_Multi/multirotor/Force//Moment computation/Forces and moments generated by spinning propellers/For Each Subsystem/Thrust//moment vector for each propeller (Body axes)/Cross Product/Subsystem ==
  u : Inport
  v : Inport  Port=2
  Demux : Demux  Outputs=3
  Demux1 : Demux  Outputs=3
  Mux : Mux  Inputs=3
  Product : Product
  Product1 : Product
  Product2 : Product
  Positive elements : Outport
  wires:
  Mux/1 -> Positive elements/1
  v/1 -> Demux1/1
  u/1 -> Demux/1
  Demux/2 -> Product/1
  Demux1/3 -> Product/2
  Demux/3 -> Product1/1
  Demux1/1 -> Product1/2
  Demux/1 -> Product2/1
  Demux1/2 -> Product2/2
  Product/1 -> Mux/1
  Product1/1 -> Mux/2
  Product2/1 -> Mux/3

== system Sim_Multi/multirotor/Force//Moment computation/Forces and moments generated by spinning propellers/For Each Subsystem/Thrust//moment vector for each propeller (Body axes)/Cross Product/Subsystem1 ==
  u : Inport
  v : Inport  Port=2
  Demux : Demux  Outputs=3
  Demux1 : Demux  Outputs=3
  Mux : Mux  Inputs=3
  Product : Product
  Product1 : Product
  Product2 : Product
  Negative elements : Outport
  wires:
  Mux/1 -> Negative elements/1
  v/1 -> Demux1/1
  u/1 -> Demux/1
  Product/1 -> Mux/1
  Product1/1 -> Mux/2
  Product2/1 -> Mux/3
  Demux/3 -> Product/1
  Demux1/2 -> Product/2
  Demux/1 -> Product1/1
  Demux1/3 -> Product1/2
  Demux/2 -> Product2/1
  Demux1/1 -> Product2/2

== system Sim_Multi/multirotor/Force//Moment computation/Compute aerodynamic drag of the airframe in Body axes/Aerodynamic drag force/Nonzero airspeed/Normalize/norm/dot_product ==
  u : Inport
  v : Inport  Port=2
  Product : Product  Multiplication=Matrix(*)  RndMeth=Zero
  Reshape : Reshape  OutputDimensionality=Column vector (2-D)
  Reshape1 : Reshape  OutputDimensionality=Column vector (2-D)
  transpose : Math  Operator=transpose  SignedPower=on
  u.v : Outport
  wires:
  v/1 -> Reshape1/1
  u/1 -> Reshape/1
  Reshape/1 -> transpose/1
  transpose/1 -> Product/1
  Reshape1/1 -> Product/2
  Product/1 -> u.v/1

== system Sim_Multi/multirotor/Force//Moment computation/Compute aerodynamic drag of the airframe in Body axes/Aerodynamic drag force/Nonzero airspeed/Surface area computation/Surface area computation/norm ==
  u : Inport
  Complex to Real-Imag : ComplexToRealImag  Output=Real
  Sqrt : Sqrt
  dot_product : Subsystem
  ||u|| : Outport
  wires:
  u/1 -> dot_product/1(u), dot_product/2(v)
  dot_product/1(u.v) -> Sqrt/1
  Sqrt/1 -> Complex to Real-Imag/1
  Complex to Real-Imag/1 -> ||u||/1

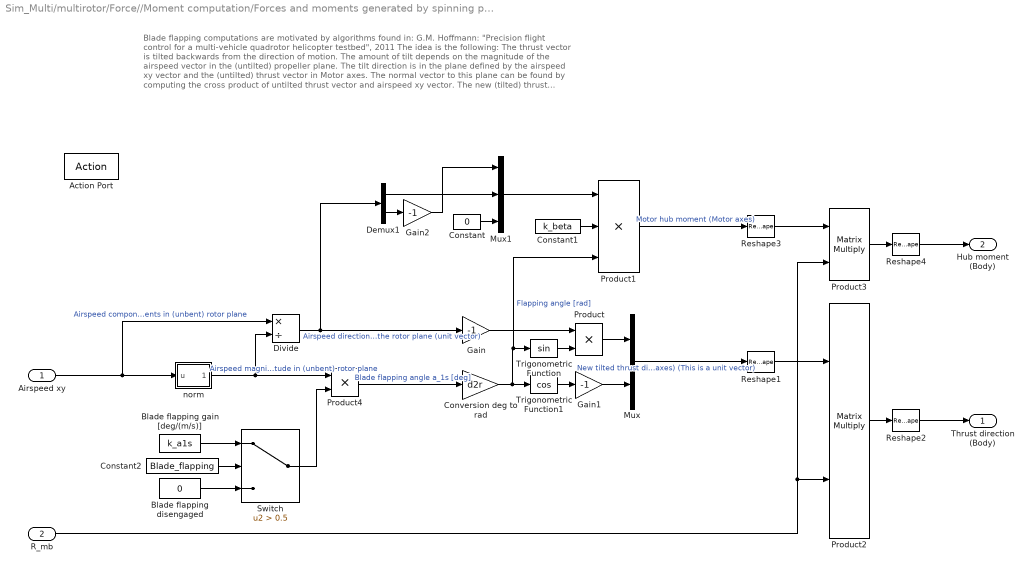
== system Sim_Multi/multirotor/Force//Moment computation/Forces and moments generated by spinning propellers/For Each Subsystem/Thrust//moment vector for each propeller (Body axes)/Compute dynamic motor thrust and moments/Blade flapping computations/Nonzero airspeed in rotor plane ==
  note: Blade flapping computations are motivated by algorithms found in:
      | G.M. Hoffmann: "Precision flight control for a multi-vehicle quadrotor helicopter testbed", 2011
      | The idea is the following:
      | The thrust vector is tilted backwards from the direction of motion. The amount of tilt depends on the magnitude of the airspeed vector in the (untilted) propeller plane.
      | The tilt direction is in the plane defined by the airspeed xy vector and the (untilted) thrust vector in Motor axes.
      | The normal vector to this plane can be found by computing the cross product of untilted thrust vector and airspeed xy vector.
      | The new (tilted) thrust vector can then be found by applying the Rodrigues rotation formula, see Wikipedia
  Airspeed xy : Inport
  R_mb : Inport  Port=2
  Action Port : ActionPort  ActionPortLabel=else
  Blade flapping disengaged : Constant  Value=0
  Blade flapping gain [deg/(m/s)] : Constant  Value=k_a1s
  Constant : Constant  Value=0
  Constant1 : Constant  Value=k_beta
  Constant2 : Constant  Value=Blade_flapping
  Conversion deg to rad : Gain  Gain=d2r
  Demux1 : Demux  Outputs=2
  Divide : Product  Inputs=*/
  Gain : Gain  Gain=-1
  Gain1 : Gain  Gain=-1
  Gain2 : Gain  Gain=-1
  Mux : Mux  Inputs=2
  Mux1 : Mux  Inputs=3
  Product : Product
  Product1 : Product  Inputs=3
  Product2 : Product  Multiplication=Matrix(*)
  Product3 : Product  Multiplication=Matrix(*)
  Product4 : Product
  Reshape1 : Reshape  OutputDimensionality=Row vector (2-D)
  Reshape2 : Reshape  OutputDimensionality=Column vector (2-D)
  Reshape3 : Reshape  OutputDimensionality=Row vector (2-D)
  Reshape4 : Reshape  OutputDimensionality=Column vector (2-D)
  Switch : Switch  Criteria=u2 > Threshold  Threshold=0.5  SaturateOnIntegerOverflow=off  InputSameDT=off
  Trigonometric Function : Trigonometry
  Trigonometric Function1 : Trigonometry  Operator=cos
  norm : Subsystem
  Thrust direction (Body) : Outport
  Hub moment (Body) : Outport  Port=2
  wires:
  Airspeed xy/1 -> Divide/1, norm/1(u)  "Airspeed components in (unbent) rotor plane"
  norm/1(||u||) -> Product4/1, Divide/2  "Airspeed magnitude in (unbent) rotor plane"
  Product4/1 -> Conversion deg to rad/1  "Blade flapping angle a_1s [deg]"
  Trigonometric Function/1 -> Product/2
  Product/1 -> Mux/1
  Trigonometric Function1/1 -> Gain1/1
  Gain1/1 -> Mux/2
  Conversion deg to rad/1 -> Product1/3, Trigonometric Function/1, Trigonometric Function1/1  "Flapping angle [rad]"
  Mux/1 -> Reshape1/1  "New tilted thrust direction vector (Motor axes) (This is a unit vector)"
  Divide/1 -> Demux1/1, Gain/1  "Airspeed direction in the rotor plane (unit vector)"
  Gain/1 -> Product/1
  Product2/1 -> Reshape2/1
  Reshape2/1 -> Thrust direction (Body)/1
  Reshape1/1 -> Product2/1
  R_mb/1 -> Product2/2, Product3/2
  Constant1/1 -> Product1/2
  Demux1/2 -> Gain2/1
  Gain2/1 -> Mux1/1
  Demux1/1 -> Mux1/2
  Constant/1 -> Mux1/3
  Mux1/1 -> Product1/1
  Product1/1 -> Reshape3/1  "Motor hub moment (Motor axes)"
  Product3/1 -> Reshape4/1
  Reshape4/1 -> Hub moment (Body)/1
  Reshape3/1 -> Product3/1
  Constant2/1 -> Switch/2
  Blade flapping gain [deg/(m/s)]/1 -> Switch/1
  Blade flapping disengaged/1 -> Switch/3
  Switch/1 -> Product4/2

== system Sim_Multi/multirotor/Force//Moment computation/Forces and moments generated by spinning propellers/For Each Subsystem/Thrust//moment vector for each propeller (Body axes)/Compute dynamic motor thrust and moments/Blade flapping computations/Zero airspeed in rotor plane ==
  Airspeed xy : Inport
  R_mb : Inport  Port=2
  Action Port : ActionPort  ActionPortLabel=if(u1 == 0)
  Constant : Constant  Value=[0;0;-1]
  Constant1 : Constant  Value=[0;0;0]
  Terminator : Terminator
  Terminator1 : Terminator
  Thrust direction (Body) : Outport  InitialOutput=[0;0;-1]
  Hub moment (Body) : Outport  Port=2  InitialOutput=[0;0;0]
  wires:
  Airspeed xy/1 -> Terminator/1  "Airspeed components in (unbent) rotor plane"
  Constant/1 -> Thrust direction (Body)/1
  Constant1/1 -> Hub moment (Body)/1
  R_mb/1 -> Terminator1/1

== system Sim_Multi/multirotor/Force//Moment computation/Forces and moments generated by spinning propellers/For Each Subsystem/Thrust//moment vector for each propeller (Body axes)/Compute dynamic motor thrust and moments/Blade flapping computations/norm ==
  u : Inport
  Complex to Real-Imag : ComplexToRealImag  Output=Real
  Sqrt : Sqrt
  dot_product : Subsystem
  ||u|| : Outport
  wires:
  u/1 -> dot_product/1(u), dot_product/2(v)
  dot_product/1(u.v) -> Sqrt/1
  Sqrt/1 -> Complex to Real-Imag/1
  Complex to Real-Imag/1 -> ||u||/1

== system Sim_Multi/multirotor/Force//Moment computation/Forces and moments generated by spinning propellers/For Each Subsystem/Thrust//moment vector for each propeller (Body axes)/Compute dynamic motor thrust and moments/Dynamic thrust ratio/Angle of attack and airspeed magnitude ==
  note: In this context, Angle of Attack is defined as zero when the airspeed lies in the propeller plane.
      | Angle of Attack increases positively when pitching up.
      | Thus, flying straight up in windless conditions would equal an AoA of -90 degrees.
      | Descending straight down in windless conditions would equal an AoA of +90 degrees.
  Airspeed (Motor axes) : Inport
  If : If  IfExpression=u1 == 0
  Merge : Merge
  Nonzero airspeed : Subsystem  TreatAsAtomicUnit=on
  Zero airspeed : Subsystem  TreatAsAtomicUnit=on
  norm2 : Subsystem
  AoA (rad) : Outport
  Airspeed magnitude : Outport  Port=2
  wires:
  If/1 -> Zero airspeed/Action
  Zero airspeed/1(AoA (rad)) -> Merge/1
  Nonzero airspeed/1(AoA (rad)) -> Merge/2
  If/2 -> Nonzero airspeed/Action
  Airspeed (Motor axes)/1 -> norm2/1(u), Nonzero airspeed/1(Airspeed (Motor)), Zero airspeed/1(Airspeed (Motor))
  Merge/1 -> AoA (rad)/1  "Angle of attack (rad)"
  norm2/1(||u||) -> Airspeed magnitude/1, If/1  "Airspeed magnitude"

== system Sim_Multi/multirotor/Force//Moment computation/Forces and moments generated by spinning propellers/For Each Subsystem/Thrust//moment vector for each propeller (Body axes)/Compute dynamic motor thrust and moments/Dynamic thrust ratio/Compute the climb speed ==
  note: This block determines the climb speed v_c
      | Since the motor coordinate system has its z-axis (along the motor axis) pointing down,
      | a positive z-velocity would mean sinking. Therefore the negative sign.
  Airspeed (Motor axes) : Inport
  Demux : Demux  Outputs=3
  Gain : Gain  Gain=-1
  Terminator : Terminator
  Terminator1 : Terminator
  v_c : Outport
  wires:
  Gain/1 -> v_c/1  "Climb speed v_c"
  Demux/1 -> Terminator/1
  Airspeed (Motor axes)/1 -> Demux/1
  Demux/2 -> Terminator1/1
  Demux/3 -> Gain/1
